simulink model "mode_calib"  (R2017a)
settings: Solver=VariableStepAuto  StartTime=0.0  StopTime=10.0  RelTol=1e-3
settings Model: Creator=Nicoe Welch  LastModifiedBy=Nicoe Welch

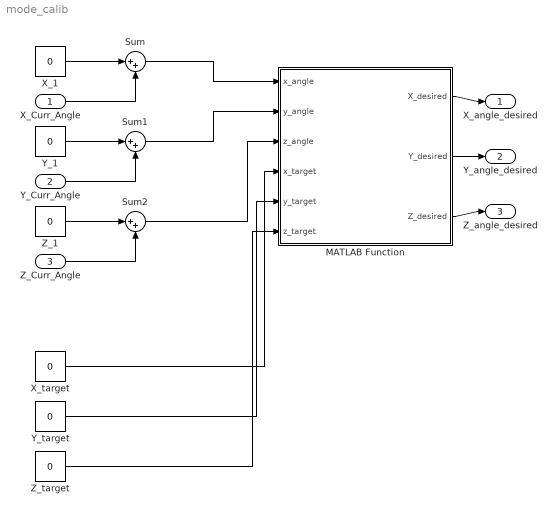
== system mode_calib ==
  X_Curr_Angle : Inport
  Y_Curr_Angle : Inport  Port=2
  Z_Curr_Angle : Inport  Port=3
  MATLAB Function : MATLAB Function  TreatAsAtomicUnit=on
  Sum : Sum  Inputs=|++
  Sum1 : Sum  Inputs=|++
  Sum2 : Sum  Inputs=|++
  X_1 : Constant  Value=0
  X_target : Constant  Value=0
  Y_1 : Constant  Value=0
  Y_target : Constant  Value=0
  Z_1 : Constant  Value=0
  Z_target : Constant  Value=0
  X_angle_desired : Outport
  Y_angle_desired : Outport  Port=2
  Z_angle_desired : Outport  Port=3
  wires:
  X_Curr_Angle/1 -> Sum/2
  X_1/1 -> Sum/1
  Y_1/1 -> Sum1/1
  Y_Curr_Angle/1 -> Sum1/2
  Z_1/1 -> Sum2/1
  Z_Curr_Angle/1 -> Sum2/2
  Sum/1 -> MATLAB Function/1(x_angle)
  Sum1/1 -> MATLAB Function/2(y_angle)
  Sum2/1 -> MATLAB Function/3(z_angle)
  X_target/1 -> MATLAB Function/4(x_target)
  Y_target/1 -> MATLAB Function/5(y_target)
  Z_target/1 -> MATLAB Function/6(z_target)
  MATLAB Function/1(X_desired) -> X_angle_desired/1
  MATLAB Function/2(Y_desired) -> Y_angle_desired/1
  MATLAB Function/3(Z_desired) -> Z_angle_desired/1

== matlab function mode_calib/MATLAB Function ==
  data: x_angle input; X_desired output; y_angle input; z_angle input; x_target input; y_target input; z_target input; Y_desired output; Z_desired output
function [X_desired, Y_desired, Z_desired] = fcn(x_angle, y_angle, z_angle, x_target, y_target, z_target)

if(x_angle ~= x_target)
    X_desired = x_target - x_angle;
else 
    if(y_angle ~= y_target)
        Y_desired = y_target - y_angle;
    else
        if(z_angle ~= z_target)
            Z_desired = z_target - z_angle;
        end
    end
end
